simulink model "cantx_0x193"  (R2022b)
settings: configuration reference "SLDD_CFG" (kept outside this file)
values from neighbouring files (symbols this model uses):
  PLCANI_APCNTL_SET_INF_2X = 0    [cantx_0x193.sldd]
  PLCANI_APCNTL_SET_INF_4X = 1    [cantx_0x193.sldd]
  PLCANI_APCNTL_SET_INF_8X = 2    [cantx_0x193.sldd]
  PLCANI_APCNTL_SET_INF_INIT = 99    [cantx_0x193.sldd]
undefined symbols (not defined in the file or in its folder): Byte0, Byte1, Byte2, Byte3, Byte4, Byte5, Byte6, Byte7
libraries: simulink x21
settings Model: DataDictionary=cantx_0x193.sldd  Creator=15801  LastModifiedBy=15801
settings ConfigSetRef: SourceName=SLDD_CFG

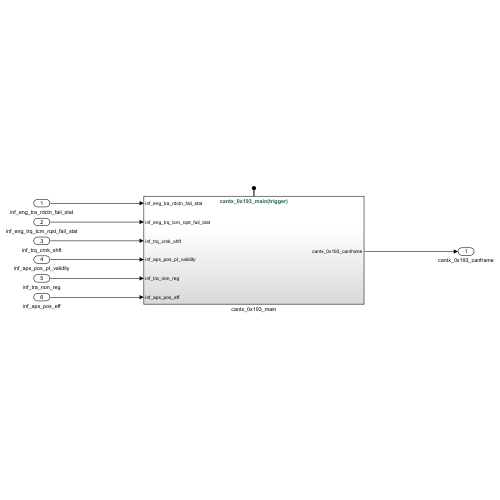
[thumbnail: Simulink's stored preview of the top-level diagram]
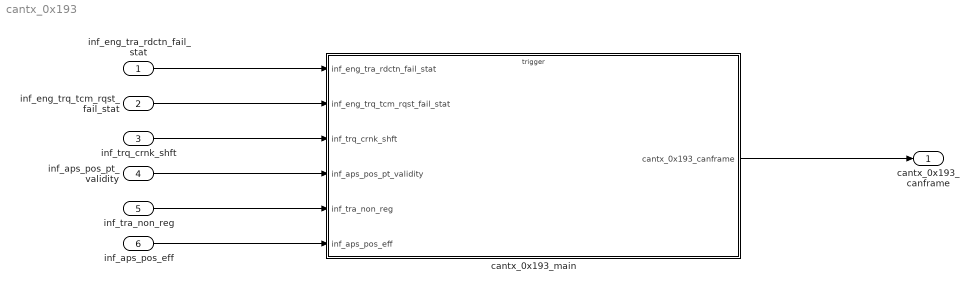
== system cantx_0x193 ==
  inf_eng_tra_rdctn_fail_stat : Inport
  inf_eng_trq_tcm_rqst_fail_stat : Inport  Port=2
  inf_trq_crnk_shft : Inport  Port=3
  inf_aps_pos_pt_validity : Inport  Port=4
  inf_tra_non_reg : Inport  Port=5
  inf_aps_pos_eff : Inport  Port=6
  cantx_0x193_main : Subsystem  TreatAsAtomicUnit=on
  cantx_0x193_canframe : Outport
  wires:
  inf_eng_tra_rdctn_fail_stat/1 -> cantx_0x193_main/1(inf_eng_tra_rdctn_fail_stat)
  inf_eng_trq_tcm_rqst_fail_stat/1 -> cantx_0x193_main/2(inf_eng_trq_tcm_rqst_fail_stat)
  inf_trq_crnk_shft/1 -> cantx_0x193_main/3(inf_trq_crnk_shft)
  inf_aps_pos_pt_validity/1 -> cantx_0x193_main/4(inf_aps_pos_pt_validity)
  inf_tra_non_reg/1 -> cantx_0x193_main/5(inf_tra_non_reg)
  inf_aps_pos_eff/1 -> cantx_0x193_main/6(inf_aps_pos_eff)
  cantx_0x193_main/1(cantx_0x193_canframe) -> cantx_0x193_canframe/1

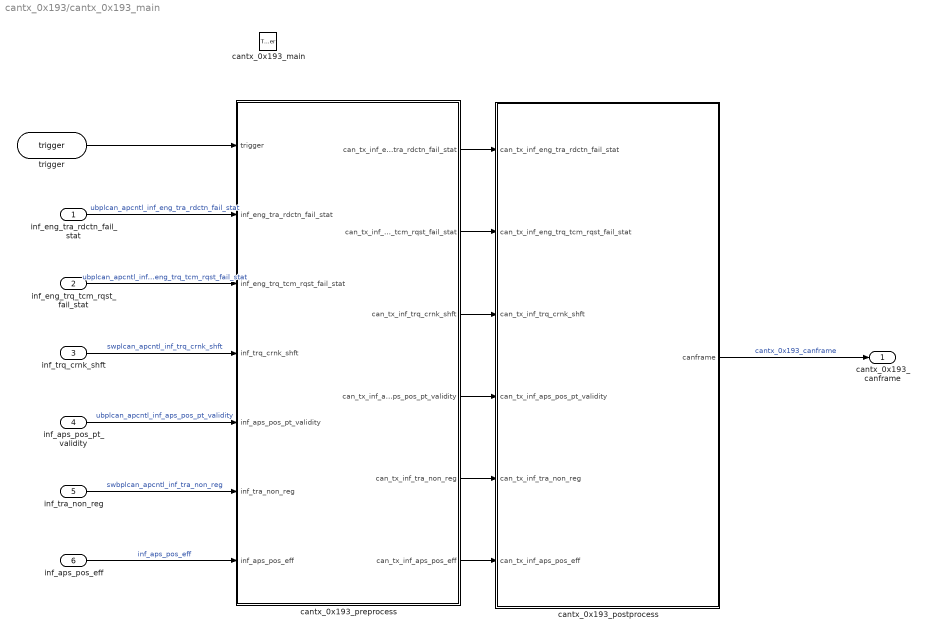
== system cantx_0x193/cantx_0x193_main ==
  inf_eng_tra_rdctn_fail_stat : Inport
  inf_eng_trq_tcm_rqst_fail_stat : Inport  Port=2
  inf_trq_crnk_shft : Inport  Port=3
  inf_aps_pos_pt_validity : Inport  Port=4
  inf_tra_non_reg : Inport  Port=5
  inf_aps_pos_eff : Inport  Port=6
  cantx_0x193_main : TriggerPort  TriggerType=function-call  IsSimulinkFunction=on  FunctionName=cantx_0x193_main  FunctionVisibility=scoped  VariantControl=(inherit)
  cantx_0x193_postprocess : Subsystem
  cantx_0x193_preprocess : Subsystem
  trigger : ArgIn  DisableCoverage=on  OutDataTypeStr=Enum: PLCANI_APCNTL_SET_INF_TYPE  ArgumentName=trigger
  cantx_0x193_canframe : Outport
  wires:
  trigger/1 -> cantx_0x193_preprocess/1(trigger)
  cantx_0x193_preprocess/1(can_tx_inf_eng_tra_rdctn_fail_stat) -> cantx_0x193_postprocess/1(can_tx_inf_eng_tra_rdctn_fail_stat)
  cantx_0x193_preprocess/2(can_tx_inf_eng_trq_tcm_rqst_fail_stat) -> cantx_0x193_postprocess/2(can_tx_inf_eng_trq_tcm_rqst_fail_stat)
  cantx_0x193_preprocess/3(can_tx_inf_trq_crnk_shft) -> cantx_0x193_postprocess/3(can_tx_inf_trq_crnk_shft)
  cantx_0x193_preprocess/4(can_tx_inf_aps_pos_pt_validity) -> cantx_0x193_postprocess/4(can_tx_inf_aps_pos_pt_validity)
  cantx_0x193_preprocess/5(can_tx_inf_tra_non_reg) -> cantx_0x193_postprocess/5(can_tx_inf_tra_non_reg)
  cantx_0x193_preprocess/6(can_tx_inf_aps_pos_eff) -> cantx_0x193_postprocess/6(can_tx_inf_aps_pos_eff)
  inf_eng_tra_rdctn_fail_stat/1 -> cantx_0x193_preprocess/2(inf_eng_tra_rdctn_fail_stat)  "ubplcan_apcntl_inf_eng_tra_rdctn_fail_stat"
  inf_eng_trq_tcm_rqst_fail_stat/1 -> cantx_0x193_preprocess/3(inf_eng_trq_tcm_rqst_fail_stat)  "ubplcan_apcntl_inf_eng_trq_tcm_rqst_fail_stat"
  inf_trq_crnk_shft/1 -> cantx_0x193_preprocess/4(inf_trq_crnk_shft)  "swplcan_apcntl_inf_trq_crnk_shft"
  inf_aps_pos_pt_validity/1 -> cantx_0x193_preprocess/5(inf_aps_pos_pt_validity)  "ubplcan_apcntl_inf_aps_pos_pt_validity"
  inf_tra_non_reg/1 -> cantx_0x193_preprocess/6(inf_tra_non_reg)  "swbplcan_apcntl_inf_tra_non_reg"
  inf_aps_pos_eff/1 -> cantx_0x193_preprocess/7(inf_aps_pos_eff)  "inf_aps_pos_eff"
  cantx_0x193_postprocess/1(canframe) -> cantx_0x193_canframe/1  "cantx_0x193_canframe"

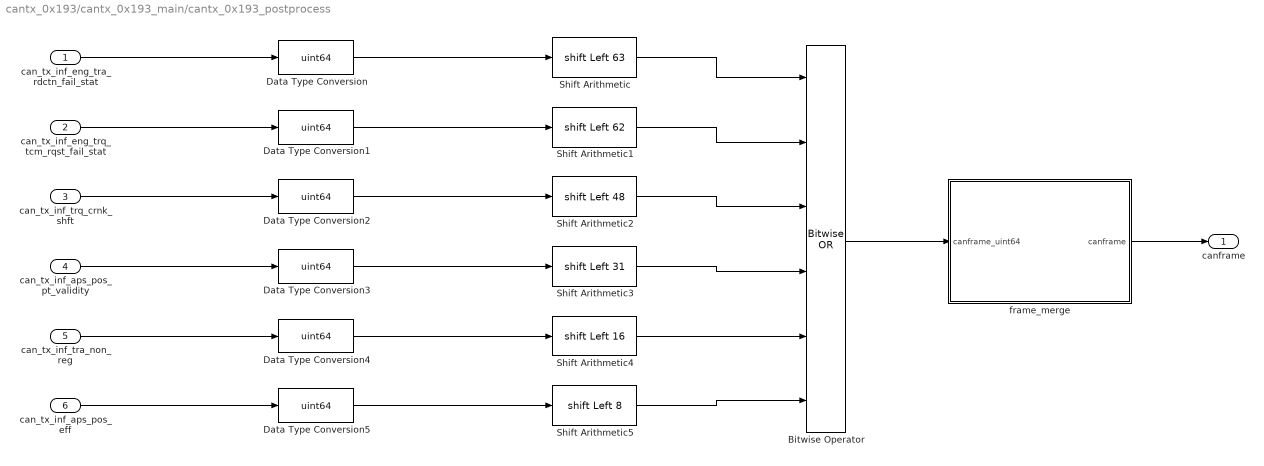
== system cantx_0x193/cantx_0x193_main/cantx_0x193_postprocess ==
  can_tx_inf_eng_tra_rdctn_fail_stat : Inport
  can_tx_inf_eng_trq_tcm_rqst_fail_stat : Inport  Port=2
  can_tx_inf_trq_crnk_shft : Inport  Port=3
  can_tx_inf_aps_pos_pt_validity : Inport  Port=4
  can_tx_inf_tra_non_reg : Inport  Port=5
  can_tx_inf_aps_pos_eff : Inport  Port=6
  Bitwise Operator : simulink/Logic and Bit Operations/Bitwise Operator  logicop=OR  UseBitMask=off  NumInputPorts=6  BitMask=bin2dec('11011001')  BitMaskRealWorld=Stored Integer
  Data Type Conversion{,1..5} (6 alike) : DataTypeConversion  OutDataTypeStr=uint64  SaturateOnIntegerOverflow=off  RndMeth=Floor
  Shift Arithmetic : ArithShift  BitShiftNumber=63  BitShiftDirection=Left
  Shift Arithmetic1 : ArithShift  BitShiftNumber=62  BitShiftDirection=Left
  Shift Arithmetic2 : ArithShift  BitShiftNumber=48  BitShiftDirection=Left
  Shift Arithmetic3 : ArithShift  BitShiftNumber=31  BitShiftDirection=Left
  Shift Arithmetic4 : ArithShift  BitShiftNumber=16  BitShiftDirection=Left
  Shift Arithmetic5 : ArithShift  BitShiftNumber=8  BitShiftDirection=Left
  frame_merge : Subsystem
  canframe : Outport
  wires:
  can_tx_inf_eng_tra_rdctn_fail_stat/1 -> Data Type Conversion/1
  Data Type Conversion/1 -> Shift Arithmetic/1
  Shift Arithmetic/1 -> Bitwise Operator/1
  can_tx_inf_eng_trq_tcm_rqst_fail_stat/1 -> Data Type Conversion1/1
  Data Type Conversion1/1 -> Shift Arithmetic1/1
  Shift Arithmetic1/1 -> Bitwise Operator/2
  can_tx_inf_trq_crnk_shft/1 -> Data Type Conversion2/1
  Data Type Conversion2/1 -> Shift Arithmetic2/1
  Shift Arithmetic2/1 -> Bitwise Operator/3
  can_tx_inf_aps_pos_pt_validity/1 -> Data Type Conversion3/1
  Data Type Conversion3/1 -> Shift Arithmetic3/1
  Shift Arithmetic3/1 -> Bitwise Operator/4
  can_tx_inf_tra_non_reg/1 -> Data Type Conversion4/1
  Data Type Conversion4/1 -> Shift Arithmetic4/1
  Shift Arithmetic4/1 -> Bitwise Operator/5
  can_tx_inf_aps_pos_eff/1 -> Data Type Conversion5/1
  Data Type Conversion5/1 -> Shift Arithmetic5/1
  Shift Arithmetic5/1 -> Bitwise Operator/6
  Bitwise Operator/1 -> frame_merge/1(canframe_uint64)
  frame_merge/1(canframe) -> canframe/1

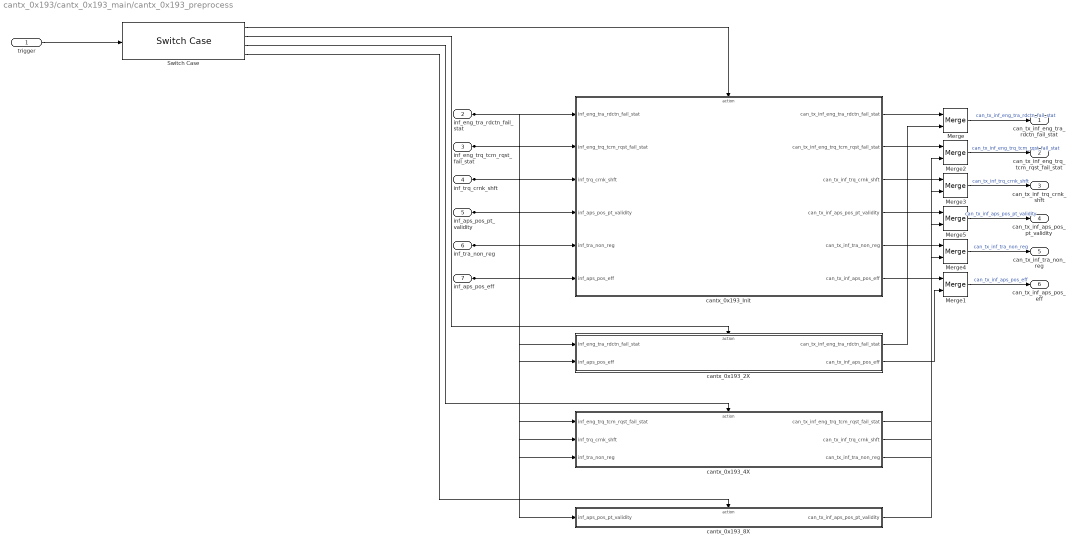
== system cantx_0x193/cantx_0x193_main/cantx_0x193_preprocess ==
  trigger : Inport
  inf_eng_tra_rdctn_fail_stat : Inport  Port=2
  inf_eng_trq_tcm_rqst_fail_stat : Inport  Port=3
  inf_trq_crnk_shft : Inport  Port=4
  inf_aps_pos_pt_validity : Inport  Port=5
  inf_tra_non_reg : Inport  Port=6
  inf_aps_pos_eff : Inport  Port=7
  Merge{,1..5} (6 alike) : Merge
  Switch Case : SwitchCase  CaseConditions={PLCANI_APCNTL_SET_INF_TYPE.PLCANI_APCNTL_SET_INF_INIT,PLCANI_APCNTL_SET_INF_TYPE.PLCANI_APCNTL_SET_INF_2X,PLCANI_APCNTL_SET_INF_TYPE.PLCANI_APCNTL_SET_INF_4X,PLCANI_APCNTL_SET_INF_TYPE.PLCANI_APCNTL_SET_INF_8X}  ShowDefaultCase=off
  cantx_0x193_2X : Subsystem  TreatAsAtomicUnit=on
      settings: RTWFcnNameOpts=Use subsystem name
  cantx_0x193_4X : Subsystem  TreatAsAtomicUnit=on
      settings: RTWFcnNameOpts=Use subsystem name
  cantx_0x193_8X : Subsystem  TreatAsAtomicUnit=on
      settings: RTWFcnNameOpts=Use subsystem name
  cantx_0x193_Init : Subsystem  TreatAsAtomicUnit=on
      settings: RTWFcnNameOpts=Use subsystem name
  can_tx_inf_eng_tra_rdctn_fail_stat : Outport
  can_tx_inf_eng_trq_tcm_rqst_fail_stat : Outport  Port=2
  can_tx_inf_trq_crnk_shft : Outport  Port=3
  can_tx_inf_aps_pos_pt_validity : Outport  Port=4
  can_tx_inf_tra_non_reg : Outport  Port=5
  can_tx_inf_aps_pos_eff : Outport  Port=6
  wires:
  trigger/1 -> Switch Case/1
  Switch Case/1 -> cantx_0x193_Init/Action
  inf_eng_tra_rdctn_fail_stat/1 -> cantx_0x193_Init/1(inf_eng_tra_rdctn_fail_stat), cantx_0x193_2X/1(inf_eng_tra_rdctn_fail_stat)
  inf_eng_trq_tcm_rqst_fail_stat/1 -> cantx_0x193_Init/2(inf_eng_trq_tcm_rqst_fail_stat), cantx_0x193_4X/1(inf_eng_trq_tcm_rqst_fail_stat)
  inf_trq_crnk_shft/1 -> cantx_0x193_Init/3(inf_trq_crnk_shft), cantx_0x193_4X/2(inf_trq_crnk_shft)
  inf_aps_pos_pt_validity/1 -> cantx_0x193_Init/4(inf_aps_pos_pt_validity), cantx_0x193_8X/1(inf_aps_pos_pt_validity)
  inf_tra_non_reg/1 -> cantx_0x193_Init/5(inf_tra_non_reg), cantx_0x193_4X/3(inf_tra_non_reg)
  inf_aps_pos_eff/1 -> cantx_0x193_Init/6(inf_aps_pos_eff), cantx_0x193_2X/2(inf_aps_pos_eff)
  Switch Case/2 -> cantx_0x193_2X/Action
  cantx_0x193_Init/1(can_tx_inf_eng_tra_rdctn_fail_stat) -> Merge/1
  cantx_0x193_2X/1(can_tx_inf_eng_tra_rdctn_fail_stat) -> Merge/2
  Merge/1 -> can_tx_inf_eng_tra_rdctn_fail_stat/1  "can_tx_inf_eng_tra_rdctn_fail_stat"
  cantx_0x193_Init/6(can_tx_inf_aps_pos_eff) -> Merge1/1
  cantx_0x193_2X/2(can_tx_inf_aps_pos_eff) -> Merge1/2
  Merge1/1 -> can_tx_inf_aps_pos_eff/1  "can_tx_inf_aps_pos_eff"
  Switch Case/3 -> cantx_0x193_4X/Action
  cantx_0x193_Init/2(can_tx_inf_eng_trq_tcm_rqst_fail_stat) -> Merge2/1
  cantx_0x193_4X/1(can_tx_inf_eng_trq_tcm_rqst_fail_stat) -> Merge2/2
  Merge2/1 -> can_tx_inf_eng_trq_tcm_rqst_fail_stat/1  "can_tx_inf_eng_trq_tcm_rqst_fail_stat"
  cantx_0x193_Init/3(can_tx_inf_trq_crnk_shft) -> Merge3/1
  cantx_0x193_4X/2(can_tx_inf_trq_crnk_shft) -> Merge3/2
  Merge3/1 -> can_tx_inf_trq_crnk_shft/1  "can_tx_inf_trq_crnk_shft"
  cantx_0x193_Init/5(can_tx_inf_tra_non_reg) -> Merge4/1
  cantx_0x193_4X/3(can_tx_inf_tra_non_reg) -> Merge4/2
  Merge4/1 -> can_tx_inf_tra_non_reg/1  "can_tx_inf_tra_non_reg"
  Switch Case/4 -> cantx_0x193_8X/Action
  cantx_0x193_Init/4(can_tx_inf_aps_pos_pt_validity) -> Merge5/1
  cantx_0x193_8X/1(can_tx_inf_aps_pos_pt_validity) -> Merge5/2
  Merge5/1 -> can_tx_inf_aps_pos_pt_validity/1  "can_tx_inf_aps_pos_pt_validity"

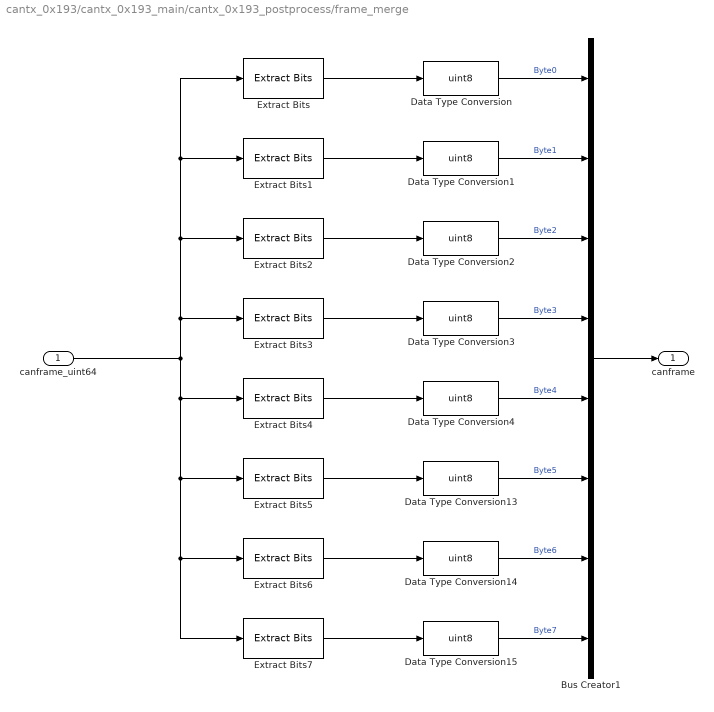
== system cantx_0x193/cantx_0x193_main/cantx_0x193_postprocess/frame_merge ==
  canframe_uint64 : Inport
  Bus Creator1 : BusCreator  Inputs=Byte0,Byte1,Byte2,Byte3,Byte4,Byte5,Byte6,Byte7  OutDataTypeStr=Bus: canframe  NonVirtualBus=on
  Data Type Conversion{,1..4,13..15} (8 alike) : DataTypeConversion  OutDataTypeStr=uint8  SaturateOnIntegerOverflow=off  RndMeth=Floor
  Extract Bits : simulink/Logic and Bit Operations/Extract Bits  bitsToExtract=Range of bits  numBits=8  bitIdxRange=[0 7]  outScalingMode=Treat bit field as an integer
  Extract Bits1 : simulink/Logic and Bit Operations/Extract Bits  bitsToExtract=Range of bits  numBits=8  bitIdxRange=[8 15]  outScalingMode=Treat bit field as an integer
  Extract Bits2 : simulink/Logic and Bit Operations/Extract Bits  bitsToExtract=Range of bits  numBits=8  bitIdxRange=[16 23]  outScalingMode=Treat bit field as an integer
  Extract Bits3 : simulink/Logic and Bit Operations/Extract Bits  bitsToExtract=Range of bits  numBits=8  bitIdxRange=[24 31]  outScalingMode=Treat bit field as an integer
  Extract Bits4 : simulink/Logic and Bit Operations/Extract Bits  bitsToExtract=Range of bits  numBits=8  bitIdxRange=[32 39]  outScalingMode=Treat bit field as an integer
  Extract Bits5 : simulink/Logic and Bit Operations/Extract Bits  bitsToExtract=Range of bits  numBits=8  bitIdxRange=[40 47]  outScalingMode=Treat bit field as an integer
  Extract Bits6 : simulink/Logic and Bit Operations/Extract Bits  bitsToExtract=Range of bits  numBits=8  bitIdxRange=[48 55]  outScalingMode=Treat bit field as an integer
  Extract Bits7 : simulink/Logic and Bit Operations/Extract Bits  bitsToExtract=Range of bits  numBits=8  bitIdxRange=[56 63]  outScalingMode=Treat bit field as an integer
  canframe : Outport
  wires:
  Bus Creator1/1 -> canframe/1
  Data Type Conversion15/1 -> Bus Creator1/8  "Byte7"
  Data Type Conversion14/1 -> Bus Creator1/7  "Byte6"
  Data Type Conversion13/1 -> Bus Creator1/6  "Byte5"
  Data Type Conversion4/1 -> Bus Creator1/5  "Byte4"
  Data Type Conversion3/1 -> Bus Creator1/4  "Byte3"
  Data Type Conversion2/1 -> Bus Creator1/3  "Byte2"
  Data Type Conversion1/1 -> Bus Creator1/2  "Byte1"
  Data Type Conversion/1 -> Bus Creator1/1  "Byte0"
  Extract Bits7/1 -> Data Type Conversion15/1
  Extract Bits6/1 -> Data Type Conversion14/1
  Extract Bits5/1 -> Data Type Conversion13/1
  Extract Bits3/1 -> Data Type Conversion3/1
  Extract Bits4/1 -> Data Type Conversion4/1
  Extract Bits2/1 -> Data Type Conversion2/1
  Extract Bits1/1 -> Data Type Conversion1/1
  Extract Bits/1 -> Data Type Conversion/1
  canframe_uint64/1 -> Extract Bits4/1, Extract Bits5/1, Extract Bits6/1, Extract Bits7/1, Extract Bits/1, Extract Bits1/1, Extract Bits2/1, Extract Bits3/1

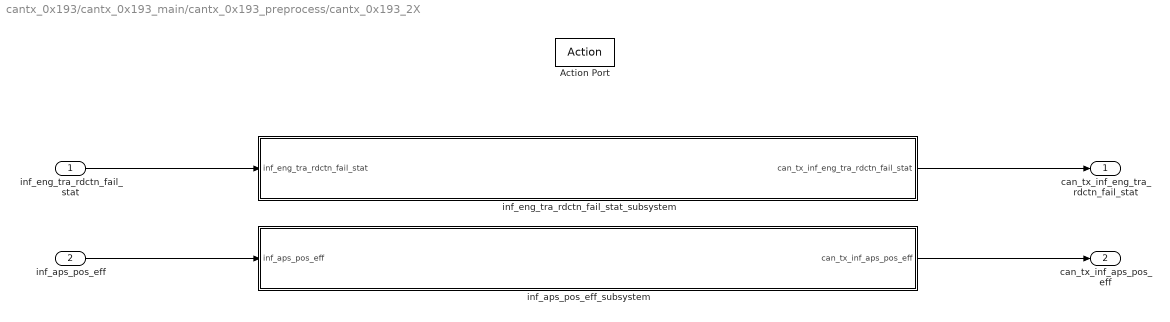
== system cantx_0x193/cantx_0x193_main/cantx_0x193_preprocess/cantx_0x193_2X ==
  inf_eng_tra_rdctn_fail_stat : Inport
  inf_aps_pos_eff : Inport  Port=2
  Action Port : ActionPort  ActionPortLabel=case [ PLCANI_APCNTL_SET_INF_2X ]:
  inf_aps_pos_eff_subsystem : Subsystem  TreatAsAtomicUnit=on
      settings: RTWFcnNameOpts=Use subsystem name
  inf_eng_tra_rdctn_fail_stat_subsystem : Subsystem  TreatAsAtomicUnit=on
      settings: RTWFcnNameOpts=Use subsystem name
  can_tx_inf_eng_tra_rdctn_fail_stat : Outport
  can_tx_inf_aps_pos_eff : Outport  Port=2
  wires:
  inf_eng_tra_rdctn_fail_stat/1 -> inf_eng_tra_rdctn_fail_stat_subsystem/1(inf_eng_tra_rdctn_fail_stat)
  inf_eng_tra_rdctn_fail_stat_subsystem/1(can_tx_inf_eng_tra_rdctn_fail_stat) -> can_tx_inf_eng_tra_rdctn_fail_stat/1
  inf_aps_pos_eff/1 -> inf_aps_pos_eff_subsystem/1(inf_aps_pos_eff)
  inf_aps_pos_eff_subsystem/1(can_tx_inf_aps_pos_eff) -> can_tx_inf_aps_pos_eff/1

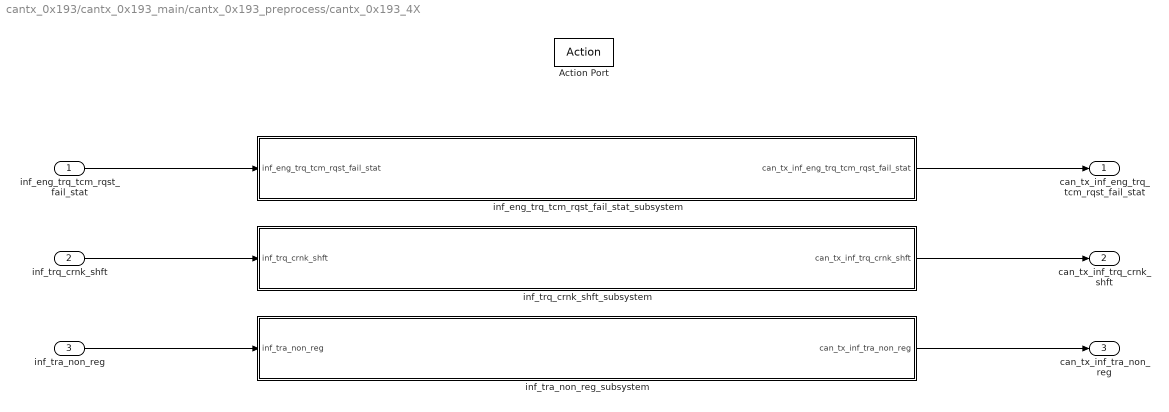
== system cantx_0x193/cantx_0x193_main/cantx_0x193_preprocess/cantx_0x193_4X ==
  inf_eng_trq_tcm_rqst_fail_stat : Inport
  inf_trq_crnk_shft : Inport  Port=2
  inf_tra_non_reg : Inport  Port=3
  Action Port : ActionPort  ActionPortLabel=case [ PLCANI_APCNTL_SET_INF_4X ]:
  inf_eng_trq_tcm_rqst_fail_stat_subsystem : Subsystem  TreatAsAtomicUnit=on
      settings: RTWFcnNameOpts=Use subsystem name
  inf_tra_non_reg_subsystem : Subsystem  TreatAsAtomicUnit=on
      settings: RTWFcnNameOpts=Use subsystem name
  inf_trq_crnk_shft_subsystem : Subsystem  TreatAsAtomicUnit=on
      settings: RTWFcnNameOpts=Use subsystem name
  can_tx_inf_eng_trq_tcm_rqst_fail_stat : Outport
  can_tx_inf_trq_crnk_shft : Outport  Port=2
  can_tx_inf_tra_non_reg : Outport  Port=3
  wires:
  inf_eng_trq_tcm_rqst_fail_stat/1 -> inf_eng_trq_tcm_rqst_fail_stat_subsystem/1(inf_eng_trq_tcm_rqst_fail_stat)
  inf_eng_trq_tcm_rqst_fail_stat_subsystem/1(can_tx_inf_eng_trq_tcm_rqst_fail_stat) -> can_tx_inf_eng_trq_tcm_rqst_fail_stat/1
  inf_trq_crnk_shft/1 -> inf_trq_crnk_shft_subsystem/1(inf_trq_crnk_shft)
  inf_trq_crnk_shft_subsystem/1(can_tx_inf_trq_crnk_shft) -> can_tx_inf_trq_crnk_shft/1
  inf_tra_non_reg/1 -> inf_tra_non_reg_subsystem/1(inf_tra_non_reg)
  inf_tra_non_reg_subsystem/1(can_tx_inf_tra_non_reg) -> can_tx_inf_tra_non_reg/1

== system cantx_0x193/cantx_0x193_main/cantx_0x193_preprocess/cantx_0x193_8X ==
  inf_aps_pos_pt_validity : Inport
  Action Port : ActionPort  ActionPortLabel=case [ PLCANI_APCNTL_SET_INF_8X ]:
  inf_aps_pos_pt_validity_subsystem : Subsystem  TreatAsAtomicUnit=on
      settings: RTWFcnNameOpts=Use subsystem name
  can_tx_inf_aps_pos_pt_validity : Outport
  wires:
  inf_aps_pos_pt_validity/1 -> inf_aps_pos_pt_validity_subsystem/1(inf_aps_pos_pt_validity)
  inf_aps_pos_pt_validity_subsystem/1(can_tx_inf_aps_pos_pt_validity) -> can_tx_inf_aps_pos_pt_validity/1

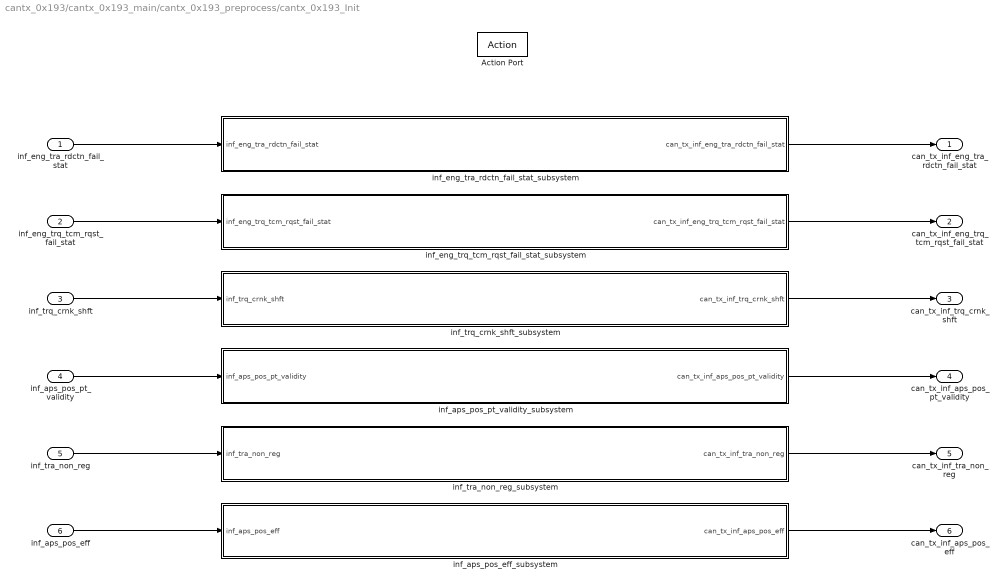
== system cantx_0x193/cantx_0x193_main/cantx_0x193_preprocess/cantx_0x193_Init ==
  inf_eng_tra_rdctn_fail_stat : Inport
  inf_eng_trq_tcm_rqst_fail_stat : Inport  Port=2
  inf_trq_crnk_shft : Inport  Port=3
  inf_aps_pos_pt_validity : Inport  Port=4
  inf_tra_non_reg : Inport  Port=5
  inf_aps_pos_eff : Inport  Port=6
  Action Port : ActionPort  ActionPortLabel=case [ PLCANI_APCNTL_SET_INF_INIT ]:
  inf_aps_pos_eff_subsystem : Subsystem  TreatAsAtomicUnit=on
      settings: RTWFcnNameOpts=Use subsystem name
  inf_aps_pos_pt_validity_subsystem : Subsystem  TreatAsAtomicUnit=on
      settings: RTWFcnNameOpts=Use subsystem name
  inf_eng_tra_rdctn_fail_stat_subsystem : Subsystem  TreatAsAtomicUnit=on
      settings: RTWFcnNameOpts=Use subsystem name
  inf_eng_trq_tcm_rqst_fail_stat_subsystem : Subsystem  TreatAsAtomicUnit=on
      settings: RTWFcnNameOpts=Use subsystem name
  inf_tra_non_reg_subsystem : Subsystem  TreatAsAtomicUnit=on
      settings: RTWFcnNameOpts=Use subsystem name
  inf_trq_crnk_shft_subsystem : Subsystem  TreatAsAtomicUnit=on
      settings: RTWFcnNameOpts=Use subsystem name
  can_tx_inf_eng_tra_rdctn_fail_stat : Outport
  can_tx_inf_eng_trq_tcm_rqst_fail_stat : Outport  Port=2
  can_tx_inf_trq_crnk_shft : Outport  Port=3
  can_tx_inf_aps_pos_pt_validity : Outport  Port=4
  can_tx_inf_tra_non_reg : Outport  Port=5
  can_tx_inf_aps_pos_eff : Outport  Port=6
  wires:
  inf_eng_tra_rdctn_fail_stat/1 -> inf_eng_tra_rdctn_fail_stat_subsystem/1(inf_eng_tra_rdctn_fail_stat)
  inf_eng_tra_rdctn_fail_stat_subsystem/1(can_tx_inf_eng_tra_rdctn_fail_stat) -> can_tx_inf_eng_tra_rdctn_fail_stat/1
  inf_eng_trq_tcm_rqst_fail_stat/1 -> inf_eng_trq_tcm_rqst_fail_stat_subsystem/1(inf_eng_trq_tcm_rqst_fail_stat)
  inf_eng_trq_tcm_rqst_fail_stat_subsystem/1(can_tx_inf_eng_trq_tcm_rqst_fail_stat) -> can_tx_inf_eng_trq_tcm_rqst_fail_stat/1
  inf_trq_crnk_shft/1 -> inf_trq_crnk_shft_subsystem/1(inf_trq_crnk_shft)
  inf_trq_crnk_shft_subsystem/1(can_tx_inf_trq_crnk_shft) -> can_tx_inf_trq_crnk_shft/1
  inf_aps_pos_pt_validity/1 -> inf_aps_pos_pt_validity_subsystem/1(inf_aps_pos_pt_validity)
  inf_aps_pos_pt_validity_subsystem/1(can_tx_inf_aps_pos_pt_validity) -> can_tx_inf_aps_pos_pt_validity/1
  inf_tra_non_reg/1 -> inf_tra_non_reg_subsystem/1(inf_tra_non_reg)
  inf_tra_non_reg_subsystem/1(can_tx_inf_tra_non_reg) -> can_tx_inf_tra_non_reg/1
  inf_aps_pos_eff/1 -> inf_aps_pos_eff_subsystem/1(inf_aps_pos_eff)
  inf_aps_pos_eff_subsystem/1(can_tx_inf_aps_pos_eff) -> can_tx_inf_aps_pos_eff/1

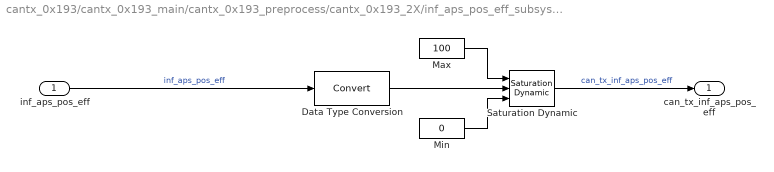
== system cantx_0x193/cantx_0x193_main/cantx_0x193_preprocess/cantx_0x193_2X/inf_aps_pos_eff_subsystem ==
  inf_aps_pos_eff : Inport
  Data Type Conversion : DataTypeConversion  SaturateOnIntegerOverflow=off  RndMeth=Floor
  Max : Constant  Value=100  OutDataTypeStr=Inherit: Inherit via back propagation
  Min : Constant  Value=0  OutDataTypeStr=Inherit: Inherit via back propagation
  Saturation Dynamic : simulink/Discontinuities/Saturation Dynamic  OutMin=[]  OutMax=[]  OutDataTypeStr=Inherit: Same as second input  OutDataType=fixdt(1, 16)  OutScaling=2^-10  DoSatur=off
  can_tx_inf_aps_pos_eff : Outport
  wires:
  Saturation Dynamic/1 -> can_tx_inf_aps_pos_eff/1  "can_tx_inf_aps_pos_eff"
  Data Type Conversion/1 -> Saturation Dynamic/2
  inf_aps_pos_eff/1 -> Data Type Conversion/1  "inf_aps_pos_eff"
  Min/1 -> Saturation Dynamic/3
  Max/1 -> Saturation Dynamic/1

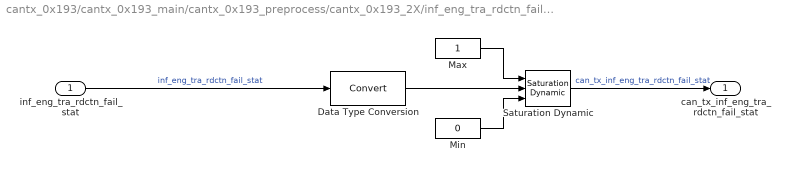
== system cantx_0x193/cantx_0x193_main/cantx_0x193_preprocess/cantx_0x193_2X/inf_eng_tra_rdctn_fail_stat_subsystem ==
  inf_eng_tra_rdctn_fail_stat : Inport
  Data Type Conversion : DataTypeConversion  SaturateOnIntegerOverflow=off  RndMeth=Floor
  Max : Constant  OutDataTypeStr=Inherit: Inherit via back propagation
  Min : Constant  Value=0  OutDataTypeStr=Inherit: Inherit via back propagation
  Saturation Dynamic : simulink/Discontinuities/Saturation Dynamic  OutMin=[]  OutMax=[]  OutDataTypeStr=Inherit: Same as second input  OutDataType=fixdt(1, 16)  OutScaling=2^-10  DoSatur=off
  can_tx_inf_eng_tra_rdctn_fail_stat : Outport
  wires:
  Saturation Dynamic/1 -> can_tx_inf_eng_tra_rdctn_fail_stat/1  "can_tx_inf_eng_tra_rdctn_fail_stat"
  Data Type Conversion/1 -> Saturation Dynamic/2
  inf_eng_tra_rdctn_fail_stat/1 -> Data Type Conversion/1  "inf_eng_tra_rdctn_fail_stat"
  Min/1 -> Saturation Dynamic/3
  Max/1 -> Saturation Dynamic/1

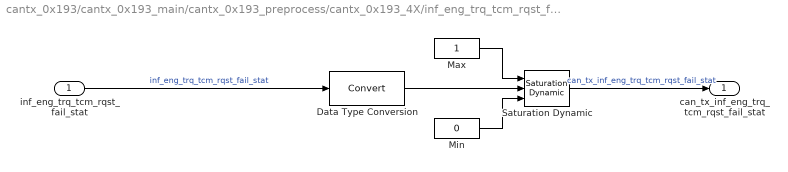
== system cantx_0x193/cantx_0x193_main/cantx_0x193_preprocess/cantx_0x193_4X/inf_eng_trq_tcm_rqst_fail_stat_subsystem ==
  inf_eng_trq_tcm_rqst_fail_stat : Inport
  Data Type Conversion : DataTypeConversion  SaturateOnIntegerOverflow=off  RndMeth=Floor
  Max : Constant  OutDataTypeStr=Inherit: Inherit via back propagation
  Min : Constant  Value=0  OutDataTypeStr=Inherit: Inherit via back propagation
  Saturation Dynamic : simulink/Discontinuities/Saturation Dynamic  OutMin=[]  OutMax=[]  OutDataTypeStr=Inherit: Same as second input  OutDataType=fixdt(1, 16)  OutScaling=2^-10  DoSatur=off
  can_tx_inf_eng_trq_tcm_rqst_fail_stat : Outport
  wires:
  Saturation Dynamic/1 -> can_tx_inf_eng_trq_tcm_rqst_fail_stat/1  "can_tx_inf_eng_trq_tcm_rqst_fail_stat"
  Data Type Conversion/1 -> Saturation Dynamic/2
  inf_eng_trq_tcm_rqst_fail_stat/1 -> Data Type Conversion/1  "inf_eng_trq_tcm_rqst_fail_stat"
  Min/1 -> Saturation Dynamic/3
  Max/1 -> Saturation Dynamic/1

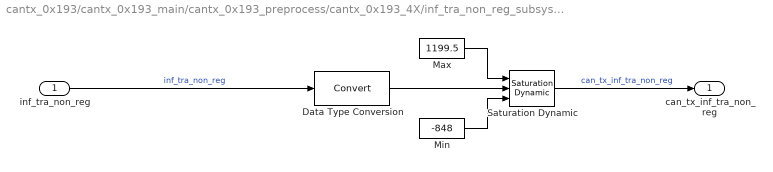
== system cantx_0x193/cantx_0x193_main/cantx_0x193_preprocess/cantx_0x193_4X/inf_tra_non_reg_subsystem ==
  inf_tra_non_reg : Inport
  Data Type Conversion : DataTypeConversion  SaturateOnIntegerOverflow=off  RndMeth=Floor
  Max : Constant  Value=1199.5  OutDataTypeStr=Inherit: Inherit via back propagation
  Min : Constant  Value=-848  OutDataTypeStr=Inherit: Inherit via back propagation
  Saturation Dynamic : simulink/Discontinuities/Saturation Dynamic  OutMin=[]  OutMax=[]  OutDataTypeStr=Inherit: Same as second input  OutDataType=fixdt(1, 16)  OutScaling=2^-10  DoSatur=off
  can_tx_inf_tra_non_reg : Outport
  wires:
  Saturation Dynamic/1 -> can_tx_inf_tra_non_reg/1  "can_tx_inf_tra_non_reg"
  Data Type Conversion/1 -> Saturation Dynamic/2
  inf_tra_non_reg/1 -> Data Type Conversion/1  "inf_tra_non_reg"
  Min/1 -> Saturation Dynamic/3
  Max/1 -> Saturation Dynamic/1

== system cantx_0x193/cantx_0x193_main/cantx_0x193_preprocess/cantx_0x193_4X/inf_trq_crnk_shft_subsystem ==
  inf_trq_crnk_shft : Inport
  Data Type Conversion : DataTypeConversion  SaturateOnIntegerOverflow=off  RndMeth=Floor
  Max : Constant  Value=1199.5  OutDataTypeStr=Inherit: Inherit via back propagation
  Min : Constant  Value=-848  OutDataTypeStr=Inherit: Inherit via back propagation
  Saturation Dynamic : simulink/Discontinuities/Saturation Dynamic  OutMin=[]  OutMax=[]  OutDataTypeStr=Inherit: Same as second input  OutDataType=fixdt(1, 16)  OutScaling=2^-10  DoSatur=off
  can_tx_inf_trq_crnk_shft : Outport
  wires:
  Saturation Dynamic/1 -> can_tx_inf_trq_crnk_shft/1  "can_tx_inf_trq_crnk_shft"
  Data Type Conversion/1 -> Saturation Dynamic/2
  inf_trq_crnk_shft/1 -> Data Type Conversion/1  "inf_trq_crnk_shft"
  Min/1 -> Saturation Dynamic/3
  Max/1 -> Saturation Dynamic/1

== system cantx_0x193/cantx_0x193_main/cantx_0x193_preprocess/cantx_0x193_8X/inf_aps_pos_pt_validity_subsystem ==
  inf_aps_pos_pt_validity : Inport
  Data Type Conversion : DataTypeConversion  SaturateOnIntegerOverflow=off  RndMeth=Floor
  Max : Constant  OutDataTypeStr=Inherit: Inherit via back propagation
  Min : Constant  Value=0  OutDataTypeStr=Inherit: Inherit via back propagation
  Saturation Dynamic : simulink/Discontinuities/Saturation Dynamic  OutMin=[]  OutMax=[]  OutDataTypeStr=Inherit: Same as second input  OutDataType=fixdt(1, 16)  OutScaling=2^-10  DoSatur=off
  can_tx_inf_aps_pos_pt_validity : Outport
  wires:
  Saturation Dynamic/1 -> can_tx_inf_aps_pos_pt_validity/1  "can_tx_inf_aps_pos_pt_validity"
  Data Type Conversion/1 -> Saturation Dynamic/2
  inf_aps_pos_pt_validity/1 -> Data Type Conversion/1  "inf_aps_pos_pt_validity"
  Min/1 -> Saturation Dynamic/3
  Max/1 -> Saturation Dynamic/1

== system cantx_0x193/cantx_0x193_main/cantx_0x193_preprocess/cantx_0x193_Init/inf_aps_pos_eff_subsystem ==
  inf_aps_pos_eff : Inport
  Data Type Conversion : DataTypeConversion  SaturateOnIntegerOverflow=off  RndMeth=Floor
  Max : Constant  Value=100  OutDataTypeStr=Inherit: Inherit via back propagation
  Min : Constant  Value=0  OutDataTypeStr=Inherit: Inherit via back propagation
  Saturation Dynamic : simulink/Discontinuities/Saturation Dynamic  OutMin=[]  OutMax=[]  OutDataTypeStr=Inherit: Same as second input  OutDataType=fixdt(1, 16)  OutScaling=2^-10  DoSatur=off
  can_tx_inf_aps_pos_eff : Outport
  wires:
  Saturation Dynamic/1 -> can_tx_inf_aps_pos_eff/1  "can_tx_inf_aps_pos_eff"
  Data Type Conversion/1 -> Saturation Dynamic/2
  inf_aps_pos_eff/1 -> Data Type Conversion/1  "inf_aps_pos_eff"
  Min/1 -> Saturation Dynamic/3
  Max/1 -> Saturation Dynamic/1

== system cantx_0x193/cantx_0x193_main/cantx_0x193_preprocess/cantx_0x193_Init/inf_aps_pos_pt_validity_subsystem ==
  inf_aps_pos_pt_validity : Inport
  Data Type Conversion : DataTypeConversion  SaturateOnIntegerOverflow=off  RndMeth=Floor
  Max : Constant  OutDataTypeStr=Inherit: Inherit via back propagation
  Min : Constant  Value=0  OutDataTypeStr=Inherit: Inherit via back propagation
  Saturation Dynamic : simulink/Discontinuities/Saturation Dynamic  OutMin=[]  OutMax=[]  OutDataTypeStr=Inherit: Same as second input  OutDataType=fixdt(1, 16)  OutScaling=2^-10  DoSatur=off
  can_tx_inf_aps_pos_pt_validity : Outport
  wires:
  Saturation Dynamic/1 -> can_tx_inf_aps_pos_pt_validity/1  "can_tx_inf_aps_pos_pt_validity"
  Data Type Conversion/1 -> Saturation Dynamic/2
  inf_aps_pos_pt_validity/1 -> Data Type Conversion/1  "inf_aps_pos_pt_validity"
  Min/1 -> Saturation Dynamic/3
  Max/1 -> Saturation Dynamic/1

== system cantx_0x193/cantx_0x193_main/cantx_0x193_preprocess/cantx_0x193_Init/inf_eng_tra_rdctn_fail_stat_subsystem ==
  inf_eng_tra_rdctn_fail_stat : Inport
  Data Type Conversion : DataTypeConversion  SaturateOnIntegerOverflow=off  RndMeth=Floor
  Max : Constant  OutDataTypeStr=Inherit: Inherit via back propagation
  Min : Constant  Value=0  OutDataTypeStr=Inherit: Inherit via back propagation
  Saturation Dynamic : simulink/Discontinuities/Saturation Dynamic  OutMin=[]  OutMax=[]  OutDataTypeStr=Inherit: Same as second input  OutDataType=fixdt(1, 16)  OutScaling=2^-10  DoSatur=off
  can_tx_inf_eng_tra_rdctn_fail_stat : Outport
  wires:
  Saturation Dynamic/1 -> can_tx_inf_eng_tra_rdctn_fail_stat/1  "can_tx_inf_eng_tra_rdctn_fail_stat"
  Data Type Conversion/1 -> Saturation Dynamic/2
  inf_eng_tra_rdctn_fail_stat/1 -> Data Type Conversion/1  "inf_eng_tra_rdctn_fail_stat"
  Min/1 -> Saturation Dynamic/3
  Max/1 -> Saturation Dynamic/1

== system cantx_0x193/cantx_0x193_main/cantx_0x193_preprocess/cantx_0x193_Init/inf_eng_trq_tcm_rqst_fail_stat_subsystem ==
  inf_eng_trq_tcm_rqst_fail_stat : Inport
  Data Type Conversion : DataTypeConversion  SaturateOnIntegerOverflow=off  RndMeth=Floor
  Max : Constant  OutDataTypeStr=Inherit: Inherit via back propagation
  Min : Constant  Value=0  OutDataTypeStr=Inherit: Inherit via back propagation
  Saturation Dynamic : simulink/Discontinuities/Saturation Dynamic  OutMin=[]  OutMax=[]  OutDataTypeStr=Inherit: Same as second input  OutDataType=fixdt(1, 16)  OutScaling=2^-10  DoSatur=off
  can_tx_inf_eng_trq_tcm_rqst_fail_stat : Outport
  wires:
  Saturation Dynamic/1 -> can_tx_inf_eng_trq_tcm_rqst_fail_stat/1  "can_tx_inf_eng_trq_tcm_rqst_fail_stat"
  Data Type Conversion/1 -> Saturation Dynamic/2
  inf_eng_trq_tcm_rqst_fail_stat/1 -> Data Type Conversion/1  "inf_eng_trq_tcm_rqst_fail_stat"
  Min/1 -> Saturation Dynamic/3
  Max/1 -> Saturation Dynamic/1

== system cantx_0x193/cantx_0x193_main/cantx_0x193_preprocess/cantx_0x193_Init/inf_tra_non_reg_subsystem ==
  inf_tra_non_reg : Inport
  Data Type Conversion : DataTypeConversion  SaturateOnIntegerOverflow=off  RndMeth=Floor
  Max : Constant  Value=1199.5  OutDataTypeStr=Inherit: Inherit via back propagation
  Min : Constant  Value=-848  OutDataTypeStr=Inherit: Inherit via back propagation
  Saturation Dynamic : simulink/Discontinuities/Saturation Dynamic  OutMin=[]  OutMax=[]  OutDataTypeStr=Inherit: Same as second input  OutDataType=fixdt(1, 16)  OutScaling=2^-10  DoSatur=off
  can_tx_inf_tra_non_reg : Outport
  wires:
  Saturation Dynamic/1 -> can_tx_inf_tra_non_reg/1  "can_tx_inf_tra_non_reg"
  Data Type Conversion/1 -> Saturation Dynamic/2
  inf_tra_non_reg/1 -> Data Type Conversion/1  "inf_tra_non_reg"
  Min/1 -> Saturation Dynamic/3
  Max/1 -> Saturation Dynamic/1

== system cantx_0x193/cantx_0x193_main/cantx_0x193_preprocess/cantx_0x193_Init/inf_trq_crnk_shft_subsystem ==
  inf_trq_crnk_shft : Inport
  Data Type Conversion : DataTypeConversion  SaturateOnIntegerOverflow=off  RndMeth=Floor
  Max : Constant  Value=1199.5  OutDataTypeStr=Inherit: Inherit via back propagation
  Min : Constant  Value=-848  OutDataTypeStr=Inherit: Inherit via back propagation
  Saturation Dynamic : simulink/Discontinuities/Saturation Dynamic  OutMin=[]  OutMax=[]  OutDataTypeStr=Inherit: Same as second input  OutDataType=fixdt(1, 16)  OutScaling=2^-10  DoSatur=off
  can_tx_inf_trq_crnk_shft : Outport
  wires:
  Saturation Dynamic/1 -> can_tx_inf_trq_crnk_shft/1  "can_tx_inf_trq_crnk_shft"
  Data Type Conversion/1 -> Saturation Dynamic/2
  inf_trq_crnk_shft/1 -> Data Type Conversion/1  "inf_trq_crnk_shft"
  Min/1 -> Saturation Dynamic/3
  Max/1 -> Saturation Dynamic/1
